simulink model "ch7example4"  (Simulink 5.0)
settings: Solver=FixedStepDiscrete  StartTime=0.0  StopTime=20.0  FixedStep=1/10  RelTol=1e-3
libraries: dspswit3 x2, commrandsrc2 x1, simulink x1
settings Model: LastModifiedBy=shaoyubin

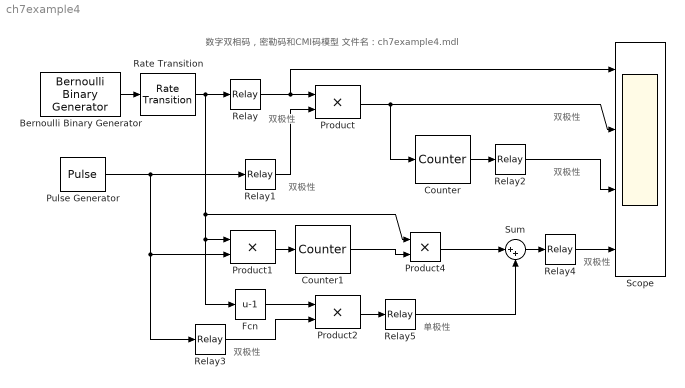
== system ch7example4 ==
  note: 数字双相码，密勒码和CMI码模型
      | 文件名：ch7example4.mdl
  note: 双极性
  note: 双极性
  note: 双极性
  note: 双极性
  note: 双极性
  note: 双极性
  note: 单极性
  Bernoulli Binary Generator : commrandsrc2/Bernoulli Binary Generator  P=0.5  seed=61  Ts=1  frameBased=off  sampPerFrame=1  orient=off
  Counter : dspswit3/Counter  Direction=Up  CountEvent=Falling edge  CounterSize=User defined  MaxCount=1  InitialCount=0  Output=Count  HitValue=32  ResetInput=off  SamplesPerFrame=1  Ts=1  CntDtype=Double  HitDtype=Logical
  Counter1 : dspswit3/Counter  Direction=Up  CountEvent=Rising edge  CounterSize=User defined  MaxCount=1  InitialCount=0  Output=Count  HitValue=32  ResetInput=off  SamplesPerFrame=1  Ts=1  CntDtype=Double  HitDtype=Logical
  Fcn : Fcn  Expr=u-1
  Product{,1..2,4} (4 alike) : Product  SaturateOnIntegerOverflow=on
  Pulse Generator : DiscretePulseGenerator  Period=10  PulseWidth=5  SampleTime=1/10
  Rate Transition : simulink/Signal Attributes/Rate Transition  DataIntegrity=on  DeterministicTransfer=on  TransitionType=Slow to fast  InitCond=0
  Relay{,1..4} (5 alike) : Relay  OnSwitchValue=0.5  OffSwitchValue=0.5  OffOutputValue=-1
  Relay5 : Relay  OnSwitchValue=0.5  OffSwitchValue=0.5
  Scope : Scope  NumInputPorts=4
      settings: TickLabels=off  YMin=-2~-2~-2~-2  YMax=2~2~2~2
  Sum : Sum  Inputs=|++  SaturateOnIntegerOverflow=on
  wires:
  Bernoulli Binary Generator/1 -> Rate Transition/1
  Rate Transition/1 -> Relay/1, Product1/1, Fcn/1, Product4/1
  Pulse Generator/1 -> Relay1/1, Product1/2, Relay3/1
  Product/1 -> Scope/2, Counter/1
  Relay/1 -> Product/1, Scope/1
  Relay1/1 -> Product/2
  Counter/1 -> Relay2/1
  Relay2/1 -> Scope/3
  Product1/1 -> Counter1/1
  Product4/1 -> Sum/1
  Fcn/1 -> Product2/1
  Product2/1 -> Relay5/1
  Sum/1 -> Relay4/1
  Relay3/1 -> Product2/2
  Relay5/1 -> Sum/2
  Counter1/1 -> Product4/2
  Relay4/1 -> Scope/4
